simulink model "Hydrostatic_Displacement_Pump"  (R2023a)
settings: Solver=VariableStepAuto  StartTime=0.0  StopTime=simtime  MaxStep=0.01  RelTol=1e-3
values from neighbouring files (symbols this model uses):
  eta_hm = 0.95    [Model_Values.mat]
  eta_vol = 0.95    [Model_Values.mat]
  J_DP = 0.02    [Model_Values.mat]
  L_FL = 0.008    [Model_Values.mat]
  M_in = 0.003    [Model_Values.mat]
  R_DP = 12    [Model_Values.mat]
  R_k = 5    [Model_Values.mat]
  R_pipe = 6    [Model_Values.mat]
  V_theo = 0.02    [Model_Values.mat]
settings Model: Creator=fycce  LastModifiedBy=fycce
settings DataIOCC: SaveOutput=off  SaveTime=off  ReturnWorkspaceOutputs=off

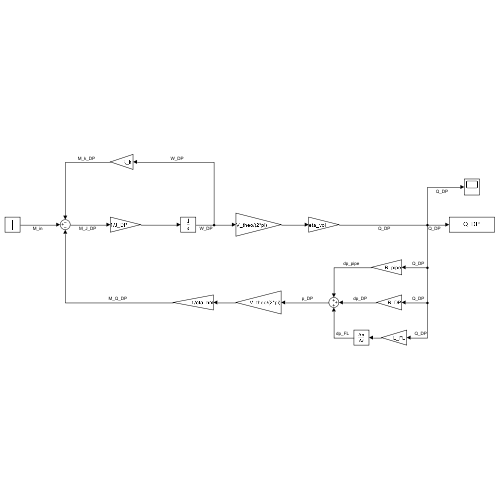
[thumbnail: Simulink's stored preview of the top-level diagram]
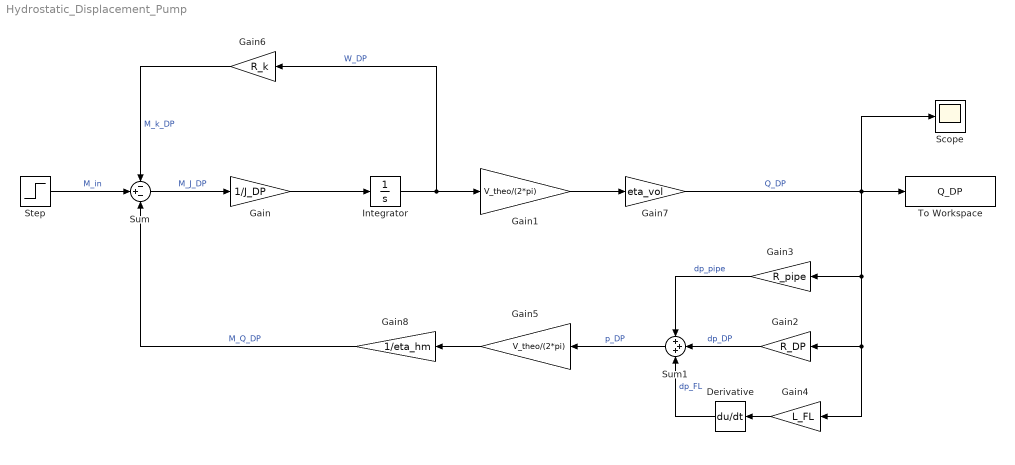
== system Hydrostatic_Displacement_Pump ==
  Derivative : Derivative
  Gain : Gain  Gain=1/J_DP
  Gain1 : Gain  Gain=V_theo/(2*pi)
  Gain2 : Gain  Gain=R_DP
  Gain3 : Gain  Gain=R_pipe
  Gain4 : Gain  Gain=L_FL
  Gain5 : Gain  Gain=V_theo/(2*pi)
  Gain6 : Gain  Gain=R_k
  Gain7 : Gain  Gain=eta_vol
  Gain8 : Gain  Gain=1/eta_hm
  Integrator : Integrator
  Scope : Scope
  Step : Step  After=M_in  SampleTime=0
  Sum : Sum  Inputs=-+-
  Sum1 : Sum  Inputs=+++
  To Workspace : ToWorkspace  VariableName=Q_DP  SaveFormat=Timeseries  SampleTime=-1
  wires:
  Step/1 -> Sum/2  "M_in"
  Sum/1 -> Gain/1  "M_J_DP"
  Gain/1 -> Integrator/1
  Integrator/1 -> Gain6/1, Gain1/1  "W_DP"
  Gain2/1 -> Sum1/2  "dp_DP"
  Gain3/1 -> Sum1/1  "dp_pipe"
  Gain4/1 -> Derivative/1
  Derivative/1 -> Sum1/3  "dp_FL"
  Gain6/1 -> Sum/1  "M_k_DP"
  Gain1/1 -> Gain7/1
  Gain7/1 -> To Workspace/1, Scope/1, Gain3/1, Gain4/1, Gain2/1  "Q_DP"
  Gain5/1 -> Gain8/1
  Sum1/1 -> Gain5/1  "p_DP"
  Gain8/1 -> Sum/3  "M_Q_DP"
